simulink model "simF16_nlinplant_unmatched"  (R2020a)
settings: Solver=ode14x  StartTime=0  StopTime=sim_t  FixedStep=Ts  RelTol=1e-3  EnableMultiTasking=on
values from neighbouring files (symbols this model uses):
  adapt_gain_no_Bm = -inv(Phi)*Mat_expm    [main_f16.m]
  Alti = A([3,5],[3,5])    [main_f16.m]
  alti_0 = sim_scenarios{i}(1)    [main_f16.m]
  altitudes = [5000 5000 5000 5000 5000 5000 5000 5000 5000 5000 5000 5000 ... (96 elements, 12x8)]    [lpv_model.mat]    (also in parameters_twoparas_ss_large_omega_range.mat)
  Ap0 = [-0.965786131048  0.940676857343; -3.44113853073  -1.30180201506]    [lpv_model.mat]    (also in parameters_twoparas_ss_large_omega_range.mat)
  Ap1 = [-0.695446741137  -0.0219021350224; -2.98749239517  -0.883673052084]    [lpv_model.mat]    (also in parameters_twoparas_ss_large_omega_range.mat)
  Ap2 = [-0.00376589285085  -0.000767161245953; 0.0864223450734  -0.00373090940113]    [lpv_model.mat]    (also in parameters_twoparas_ss_large_omega_range.mat)
  Blti = B([3,5],2)    [main_f16.m]
  Bp0 = [-0.00202220767716 -0.26458627897]    [lpv_model.mat]    (also in parameters_twoparas_ss_large_omega_range.mat)
  Bp1 = [-0.00144075289053 -0.241352628281]    [lpv_model.mat]    (also in parameters_twoparas_ss_large_omega_range.mat)
  Bp2 = [-6.1325666296e-07 -0.000135209280723]    [lpv_model.mat]    (also in parameters_twoparas_ss_large_omega_range.mat)
  control_trims = [0.149023636522 -3.3718875614 -3.81812148762e-13 -1.65140410369e-12 0.145229850722 -2.69024444853 -5.03470498061e-14 -2.84198247296e-13 0.146487538342 -2.32267253452 7.51716315972e-14 5.14334939656e-13 ... (384 elements, 4x12x8)]    [lpv_model.mat]    (also in parameters_twoparas_ss_large_omega_range.mat)
  Cp = [1 0]    [lpv_model.mat]    (also in parameters_twoparas_ss_large_omega_range.mat)
  duration = 3.01    [main_f16.m]
  enable_L1 = 1    [main_f16.m]
  enable_um_dist_comp = 1    [main_f16.m]
  L = [-1.0529546208e-07 9.01402394984e-07 -6.3448246624e-08 3.15977865752e-07 2.28928663113e-09 -4.32057794956e-09]    [parameters_twoparas_ss_large_omega_range.mat]
  opt =     [unmatched_comp_filter.mat]
  pbar_lower_bnd = 37.1201390864    [lpv_model.mat]    (also in parameters_twoparas_ss_large_omega_range.mat)
  pbar_upper_bnd = 830.356708228    [lpv_model.mat]    (also in parameters_twoparas_ss_large_omega_range.mat)
  r2d = 180/pi    (= 57.2957795131)    [main_f16.m]
  ref_step = 2    [main_f16.m]
  sample_time = Ts    (= 0.001)    [main_f16.m]
  simu_index = simu_index+1    (= 2)    [main_f16.m]
  state_trims = [350 0.128572104103 1.56844869675e-16 0 0.128572104103 0 0 0 0 0 0 5000 ... (1248 elements, 13x12x8)]    [lpv_model.mat]    (also in parameters_twoparas_ss_large_omega_range.mat)
  Ts = 1e-3    (= 0.001)    [main_f16.m]
  unknown_input_gain = .7    (= 0.7)    [main_f16.m]
  veloc_0 = sim_scenarios{i}(2)    [main_f16.m]
  veloc_max = 900    [lpv_model.mat]    (also in parameters_twoparas_ss_large_omega_range.mat)
  veloc_min = 350    [lpv_model.mat]    (also in parameters_twoparas_ss_large_omega_range.mat)
  velocities = [350 400 450 500 550 600 650 700 750 800 850 900 ... (96 elements, 12x8)]    [lpv_model.mat]    (also in parameters_twoparas_ss_large_omega_range.mat)
  X = [4.80336810738e-09 -1.50779531784e-08 -1.50779531784e-08 7.69063603425e-08 2.19210658353e-09 -1.15520629836e-08 -1.15520629836e-08 6.7948487849e-08 9.47019033424e-11 -1.37129742327e-10 -1.37129742327e-10 2.78905243689e-10]    [parameters_twoparas_ss_large_omega_range.mat]
undefined symbols (not defined in the file or in its folder): C_den, C_num, control_trim, state_trim
settings Model: ExtModeAutoUpdateStatusClock=off  Creator=keviczky  LastModifiedBy=Boran
settings DataIOCC: Decimation=50  SaveFormat=Array  SignalLoggingSaveFormat=ModelDataLogs  ReturnWorkspaceOutputs=off  SignalLoggingName=sigsOut
settings OptimizationCC: BooleanDataType=off
settings DebuggingCC: AlgebraicLoopMsg=error  SaveWithParameterizedLinksMsg=none  UnderspecifiedInitializationDetection=Classic  MergeDetectMultiDrivingBlocksExec=none  SignalResolutionControl=TryResolveAllWithWarning  MultiTaskDSMMsg=warning  MultiTaskCondExecSysMsg=none  ArithmeticOperatorsInVariantConditions=warning
settings HardwareCC: ProdBitPerPointer=32  ProdBitPerSizeT=32  ProdBitPerPtrDiffT=32  ProdLargestAtomicFloat=None  ProdIntDivRoundTo=Undefined  ProdEndianess=Unspecified  ProdWordSize=32  ProdHWDeviceType=32-bit Generic  TargetBitPerPointer=64  TargetBitPerSizeT=64  TargetBitPerPtrDiffT=64  TargetLongLongMode=on  TargetIntDivRoundTo=Zero  TargetEndianess=LittleEndian  TargetWordSize=64  TargetHWDeviceType=MATLAB Host  ProdEqTarget=off
settings ModelReferenceCC: PropagateSignalLabelsOutOfModel=off
settings SFSimCC: CustomCodeUndefinedFunction=UseInterfaceOnly
settings GRTTargetCC: CombineOutputUpdateFcns=off  GRTInterface=on
settings ConfigComp: CovMetricSettings=dw  CovHtmlReporting=on  CovSaveCumulativeToWorkspaceVar=on  CovSaveSingleToWorkspaceVar=on

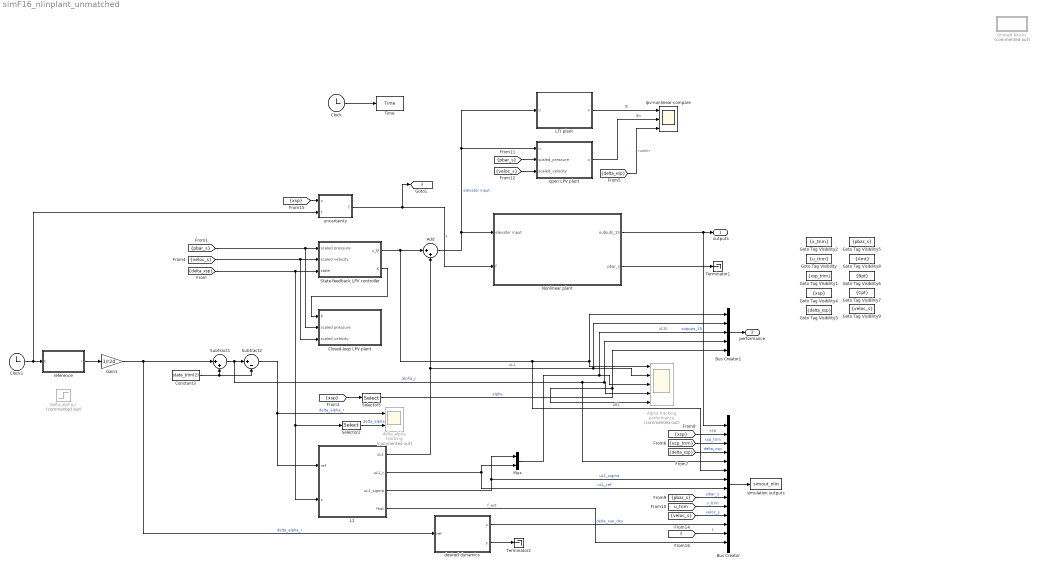
== system simF16_nlinplant_unmatched ==
  Add : Sum  Inputs=|++
  Alpha tracking performance : Scope  Commented=on  NumInputPorts=5
  Bus Creator : BusCreator  Inputs=14
  Bus Creator1 : BusCreator  Inputs=5
  Clock : Clock
      settings: Decimation=50
  Clock1 : Clock
      settings: Decimation=50
  Closed-loop LPV plant : Subsystem
  Constant3 : Constant  Value=state_trim(2)
  Gain1 : Gain  Gain=1/r2d
  Goto Tag Visibility : GotoTagVisibility  GotoTag=u_trim
  Goto Tag Visibility1 : GotoTagVisibility  GotoTag=xsp_trim
  Goto Tag Visibility2 : GotoTagVisibility  GotoTag=x_trim
  Goto Tag Visibility3 : GotoTagVisibility  GotoTag=delta_xsp
  Goto Tag Visibility4 : GotoTagVisibility  GotoTag=xsp
  Goto Tag Visibility5 : GotoTagVisibility  GotoTag=pbar_s
  Goto Tag Visibility6 : GotoTagVisibility  GotoTag=Bpt
  Goto Tag Visibility7 : GotoTagVisibility  GotoTag=Cpt
  Goto Tag Visibility8 : GotoTagVisibility  GotoTag=Amt
  Goto Tag Visibility9 : GotoTagVisibility  GotoTag=veloc_s
  "L1 " : Subsystem
  LTI plant : Subsystem
  Mux : Mux  Inputs=2
  "Nonlinear plant " : Subsystem
  Selector2 : Selector  InputPortWidth=2  IndexOptions=Index vector (dialog)  Indices=1  OutputSizes=1
  Selector5 : Selector  InputPortWidth=2  IndexOptions=Index vector (dialog)  Indices=1  OutputSizes=1
  State-feedback LPV controller : Subsystem
  Subtract1 : Sum  Inputs=|++
  Subtract2 : Sum  Inputs=|+-
  Terminator1 : Terminator
  Terminator2 : Terminator
  Time : ToWorkspace  VariableName=Time  SampleTime=-1
      settings: Decimation=100
  Unused blocks : Subsystem  Commented=on
  delta_alpha tracking : Scope  Commented=on  NumInputPorts=2
  delta_alpha_r : Step  Commented=on  SampleTime=0
  desired dynamics : Subsystem
  lpv-nonlinear-compare : Scope  NumInputPorts=3
  open LPV plant : Subsystem
  reference : MATLAB Function  TreatAsAtomicUnit=on
  simulation outputs : ToWorkspace  VariableName=simout_nlin  SaveFormat=Timeseries  SampleTime=-1
      settings: Decimation=2
  uncertainty : MATLAB Function  TreatAsAtomicUnit=on
  outputs : Outport  VectorParamsAs1DForOutWhenUnconnected=off
  performance : Outport  Port=2  VectorParamsAs1DForOutWhenUnconnected=off
  tag scope: f=global
  wires:
  Clock/1 -> Time/1
  "L1 "/4(fhat) -> Bus Creator/14  "f_est"
  [f] -> Bus Creator/13  "f"
  [delta_xsp] -> lpv-nonlinear-compare/3  "nonlin"
  uncertainty/1(f) -> "Nonlinear plant "/2(f), [f]  "f"
  open LPV plant/1(x) -> lpv-nonlinear-compare/2  "lpv"
  [pbar_s] -> open LPV plant/2(scaled_pressure)
  [delta_xsp] -> Bus Creator/4  "delta_xsp"
  Add/1 -> "Nonlinear plant "/1(elevator input), LTI plant/1(u), open LPV plant/1(u)  "elevator input"
  Clock1/1 -> uncertainty/2(t), reference/1(t)
  Bus Creator1/1 -> performance/1
  [xsp] -> uncertainty/1(x)
  desired dynamics/1(x) -> Bus Creator/12  "delta_xsp_des"
  desired dynamics/2(y) -> Terminator2/1
  [veloc_s] -> Bus Creator/11  "veloc_s"
  [xsp] -> Bus Creator/2  "xsp"
  State-feedback LPV controller/2(K) -> Closed-loop LPV plant/1(K)
  "Nonlinear plant "/1(outputs_15) -> outputs/1, Bus Creator/1  "outputs_15"
  Gain1/1 -> desired dynamics/1(ref), Subtract1/1  "delta_alpha_r"
  [veloc_s] -> open LPV plant/3(scaled_velocity)
  [xsp_trim] -> Bus Creator/3  "xsp_trim"
  LTI plant/1(x) -> lpv-nonlinear-compare/1  "lti"
  reference/1(r) -> Gain1/1
  [delta_xsp] -> State-feedback LPV controller/3(state), "L1 "/2(x), Selector2/1
  "L1 "/2(uL1_r) -> Mux/2, Bus Creator/8  "uL1_ref"
  [veloc_s] -> Closed-loop LPV plant/3(scaled velocity), State-feedback LPV controller/2(scaled velocity)
  [xsp] -> Selector5/1
  Selector2/1 -> delta_alpha tracking/2  "delta_alpha"
  Constant3/1 -> Subtract2/2, Subtract1/2
  "L1 "/1(uL1) -> Add/2, Bus Creator1/2, Alpha tracking performance/2  "uL1"
  [pbar_s] -> Bus Creator/9  "pbar_s"
  Bus Creator/1 -> simulation outputs/1
  State-feedback LPV controller/1(u_bl) -> Add/1, Bus Creator/6, Bus Creator1/1, Alpha tracking performance/1  "uBL"
  "L1 "/3(uL1_sigma) -> Mux/1, Bus Creator/7  "uL1_sigma"
  Subtract2/1 -> "L1 "/1(ref), delta_alpha tracking/1  "delta_alpha_r"
  [pbar_s] -> Closed-loop LPV plant/2(scaled pressure), State-feedback LPV controller/1(scaled pressure)
  Mux/1 -> Bus Creator1/3, Alpha tracking performance/3  "uL1s"
  Selector5/1 -> Alpha tracking performance/5, Bus Creator1/5  "alpha"
  "Nonlinear plant "/2(pbar_s) -> Terminator1/1
  Subtract1/1 -> Alpha tracking performance/4, Bus Creator1/4, Bus Creator/5, Subtract2/1  "alpha_r"
  [u_trim] -> Bus Creator/10  "u_trim"

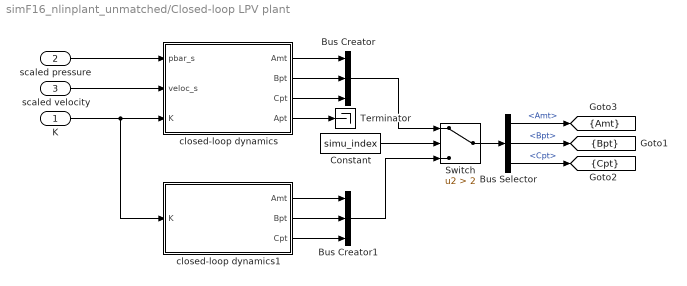
== system simF16_nlinplant_unmatched/Closed-loop LPV plant ==
  K : Inport
  scaled pressure : Inport  Port=2
  scaled velocity : Inport  Port=3
  Bus Creator : BusCreator  Inputs=3
  Bus Creator1 : BusCreator  Inputs=3
  Bus Selector : BusSelector  OutputSignals=Amt,Bpt,Cpt
  Constant : Constant  Value=simu_index
  Switch : Switch  Criteria=u2 > Threshold  Threshold=2
  Terminator : Terminator
  closed-loop dynamics : MATLAB Function  TreatAsAtomicUnit=on
  closed-loop dynamics1 : MATLAB Function  TreatAsAtomicUnit=on
  tag scope: Amt=scoped, Bpt=scoped, Cpt=scoped
  wires:
  scaled pressure/1 -> closed-loop dynamics/1(pbar_s)
  scaled velocity/1 -> closed-loop dynamics/2(veloc_s)
  closed-loop dynamics/2(Bpt) -> Bus Creator/2
  closed-loop dynamics/4(Apt) -> Terminator/1
  closed-loop dynamics/1(Amt) -> Bus Creator/1
  closed-loop dynamics/3(Cpt) -> Bus Creator/3
  closed-loop dynamics1/1(Amt) -> Bus Creator1/1
  closed-loop dynamics1/2(Bpt) -> Bus Creator1/2
  closed-loop dynamics1/3(Cpt) -> Bus Creator1/3
  Bus Creator/1 -> Switch/1
  Bus Creator1/1 -> Switch/3
  Switch/1 -> Bus Selector/1
  Bus Selector/1 -> [Amt]  "<Amt>"
  Bus Selector/2 -> [Bpt]  "<Bpt>"
  Bus Selector/3 -> [Cpt]  "<Cpt>"
  K/1 -> closed-loop dynamics1/1(K), closed-loop dynamics/3(K)
  Constant/1 -> Switch/2

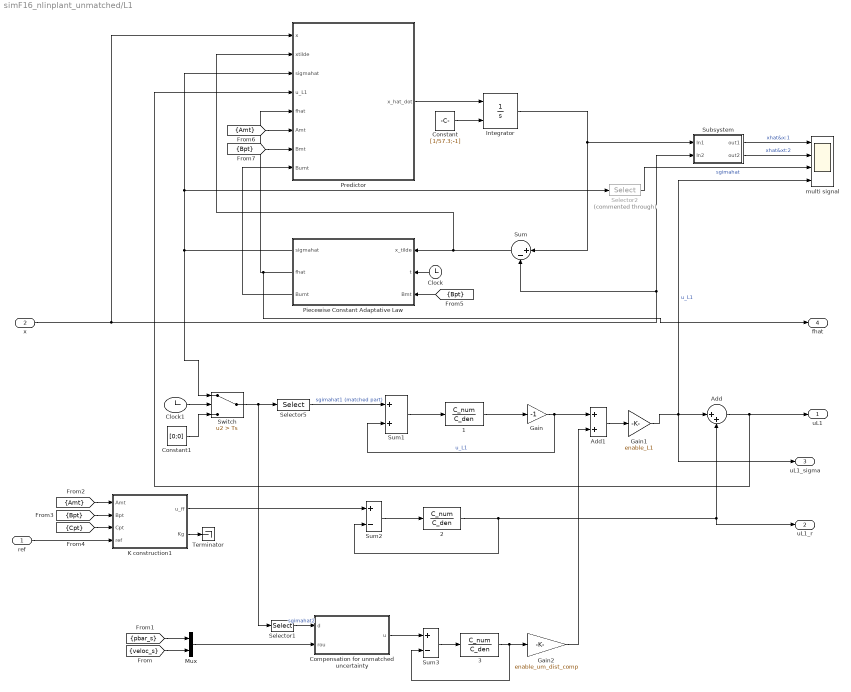
== system simF16_nlinplant_unmatched/L1  ==
  ref : Inport
  x : Inport  Port=2
  " 1" : TransferFcn  Numerator=C_num  Denominator=C_den
  " 2" : TransferFcn  Numerator=C_num  Denominator=C_den
  " 3" : TransferFcn  Numerator=C_num  Denominator=C_den
  Add : Sum  Inputs=|++
  Add1 : Sum
  Clock : Clock
  Clock1 : Clock
      settings: Decimation=50
  Compensation for unmatched uncertainty : Subsystem
  Constant : Constant  Value=[1/57.3;-1]
  Constant1 : Constant  Value=[0;0]
  Gain : Gain  Gain=-1
  Gain1 : Gain  Gain=enable_L1
  Gain2 : Gain  Gain=enable_um_dist_comp
  Integrator : Integrator  InitialConditionSource=external
  K construction1 : MATLAB Function  TreatAsAtomicUnit=on
  Mux : Mux  Inputs=2
  Piecewise Constant Adaptative Law : MATLAB Function  TreatAsAtomicUnit=on
  Predictor : MATLAB Function  TreatAsAtomicUnit=on
  Selector1 : Selector  InputPortWidth=2  IndexOptions=Index vector (dialog)  Indices=2  OutputSizes=1
  Selector2 : Selector  Commented=through  InputPortWidth=2  IndexOptions=Index vector (dialog)  Indices=[1]  OutputSizes=1
  Selector5 : Selector  InputPortWidth=2  IndexOptions=Index vector (dialog)  Indices=[1]  OutputSizes=1
  Subsystem : Subsystem
  Sum : Sum  Inputs=|+-
  Sum1 : Sum
  Sum2 : Sum  Inputs=+-
  Sum3 : Sum  Inputs=+-
  Switch : Switch  Criteria=u2 > Threshold  Threshold=Ts
  Terminator : Terminator
  "multi signal " : Scope  NumInputPorts=4
  uL1 : Outport  VectorParamsAs1DForOutWhenUnconnected=off
  uL1_r : Outport  Port=2  VectorParamsAs1DForOutWhenUnconnected=off
  uL1_sigma : Outport  Port=3  VectorParamsAs1DForOutWhenUnconnected=off
  fhat : Outport  Port=4  VectorParamsAs1DForOutWhenUnconnected=off
  wires:
  Constant/1 -> Integrator/2
  Predictor/1(x_hat_dot) -> Integrator/1
  Integrator/1 -> Sum/1, Subsystem/1(In1)
  Clock/1 -> Piecewise Constant Adaptative Law/2(t)
  x/1 -> Subsystem/2(In2), Sum/2, Predictor/1(x)
  Selector2/1 -> "multi signal "/3  "sgimahat"
  Gain1/1 -> Add/1, uL1_sigma/1, "multi signal "/4  "u_L1"
  " 1"/1 -> Gain/1
  [Cpt] -> K construction1/3(Cpt)
  [Bpt] -> K construction1/2(Bpt)
  " 2"/1 -> Add/2, uL1_r/1, Sum2/2
  ref/1 -> K construction1/4(ref)
  [Amt] -> K construction1/1(Amt)
  [Bpt] -> Piecewise Constant Adaptative Law/3(Bmt)
  [Amt] -> Predictor/6(Amt)
  [Bpt] -> Predictor/7(Bmt)
  Sum/1 -> Piecewise Constant Adaptative Law/1(x_tilde), Predictor/2(xtilde)
  Selector5/1 -> Sum1/1  "sgimahat1 (matched part)"
  Sum1/1 -> " 1"/1
  Piecewise Constant Adaptative Law/3(Bumt) -> Predictor/8(Bumt)
  Sum2/1 -> " 2"/1
  Subsystem/1(out1) -> "multi signal "/1  "xhat&x:1"
  Subsystem/2(out2) -> "multi signal "/2  "xhat&xt:2"
  Add/1 -> Predictor/4(u_L1), uL1/1
  K construction1/2(Kg) -> Terminator/1
  Gain2/1 -> Add1/2
  Mux/1 -> Compensation for unmatched uncertainty/2(rou)
  Selector1/1 -> Compensation for unmatched uncertainty/1(d)  "sgimahat2"
  [veloc_s] -> Mux/2
  Compensation for unmatched uncertainty/1(u) -> Sum3/1
  Sum3/1 -> " 3"/1
  [pbar_s] -> Mux/1
  " 3"/1 -> Gain2/1, Sum3/2
  Piecewise Constant Adaptative Law/1(sigmahat) -> Switch/1, Predictor/3(sigmahat), Selector2/1
  Add1/1 -> Gain1/1
  Gain/1 -> Sum1/2, Add1/1  "u_L1"
  Piecewise Constant Adaptative Law/2(fhat) -> fhat/1, Predictor/5(fhat)
  Constant1/1 -> Switch/3
  Switch/1 -> Selector1/1, Selector5/1
  Clock1/1 -> Switch/2
  K construction1/1(u_ff) -> Sum2/1

== system simF16_nlinplant_unmatched/LTI plant ==
  u : Inport
  Integrator : Integrator
  K construction : MATLAB Function  TreatAsAtomicUnit=on
  x : Outport  VectorParamsAs1DForOutWhenUnconnected=off
  wires:
  u/1 -> K construction/2(u)
  K construction/1(xdot) -> Integrator/1
  Integrator/1 -> x/1, K construction/1(x)

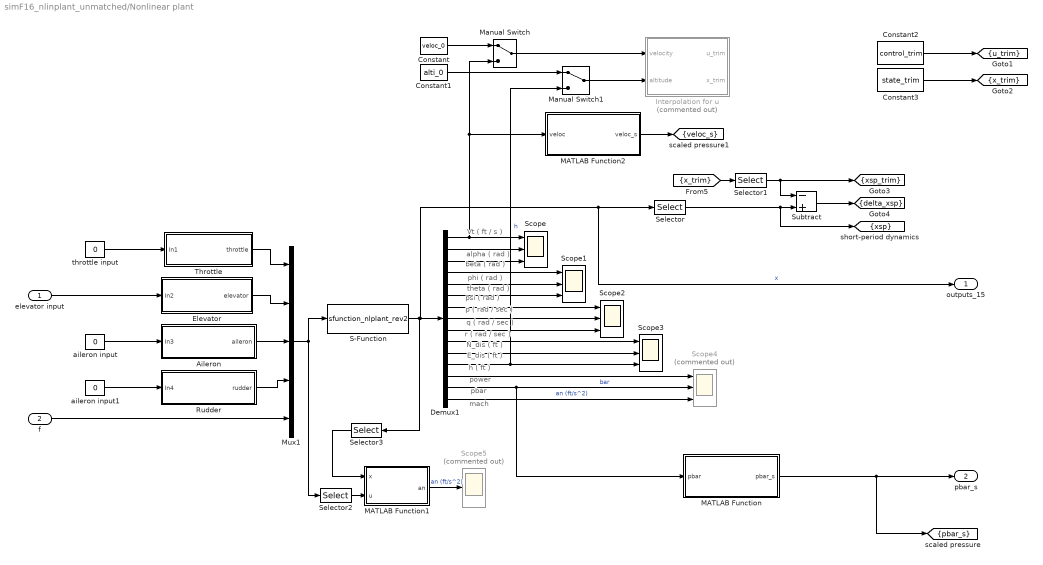
== system simF16_nlinplant_unmatched/Nonlinear plant  ==
  note: Vt ( ft / s )
  note: alpha ( rad )
  note: beta ( rad )
  note: phi ( rad )
  note: theta ( rad )
  note: psi ( rad )
  note: p ( rad / sec )
  note: q ( rad / sec )
  note: r ( rad / sec )
  note: N_dis ( ft )
  note: E_dis ( ft )
  note: h ( ft )
  note: power
  note: pbar
  note: mach
  elevator input : Inport
  f : Inport  Port=2
  Aileron : Subsystem
  Constant : Constant  Value=veloc_0
  Constant1 : Constant  Value=alti_0
  Constant2 : Constant  Value=control_trim
  Constant3 : Constant  Value=state_trim
  Demux1 : Demux  Outputs=15
  Elevator : Subsystem
  Interpolation for u : Subsystem  Commented=on
  MATLAB Function : MATLAB Function  TreatAsAtomicUnit=on
  MATLAB Function1 : MATLAB Function  TreatAsAtomicUnit=on
  MATLAB Function2 : MATLAB Function  TreatAsAtomicUnit=on
  Manual Switch : ManualSwitch
  Manual Switch1 : ManualSwitch
  Mux1 : Mux  Inputs=5
  Rudder : Subsystem
  S-Function : S-Function  FunctionName=sfunction_nlplant_rev2  Parameters="state_trim,  xcg"  SFunctionDeploymentMode=off  EnableBusSupport=off
  Scope{,1..3} (4 alike) : Scope  NumInputPorts=3
  Scope4 : Scope  Commented=on  NumInputPorts=3
  Scope5 : Scope  Commented=on
  Selector : Selector  InputPortWidth=15  IndexOptions=Index vector (dialog)  Indices=[2 8]  OutputSizes=1
  Selector1 : Selector  InputPortWidth=13  IndexOptions=Index vector (dialog)  Indices=[2 8]  OutputSizes=1
  Selector2 : Selector  InputPortWidth=6  IndexOptions=Index vector (dialog)  Indices=1:4  OutputSizes=1
  Selector3 : Selector  InputPortWidth=15  IndexOptions=Index vector (dialog)  Indices=[1:13]  OutputSizes=1
  Subtract : Sum  Inputs=-+
  Throttle : Subsystem
  aileron input : Constant  Value=0
  aileron input1 : Constant  Value=0
  throttle input : Constant  Value=0
  outputs_15 : Outport  VectorParamsAs1DForOutWhenUnconnected=off
  pbar_s : Outport  Port=2  VectorParamsAs1DForOutWhenUnconnected=off
  tag scope: delta_xsp=scoped, pbar_s=scoped, u_trim=scoped, veloc_s=scoped, x_trim=scoped, xsp=scoped, xsp_trim=scoped
  wires:
  Demux1/6 -> Scope1/3
  Demux1/7 -> Scope2/1
  Demux1/2 -> Scope/2
  Constant1/1 -> Manual Switch1/1
  Demux1/3 -> Scope/3
  aileron input1/1 -> Rudder/1(In4)
  S-Function/1 -> Selector3/1, Demux1/1, outputs_15/1, Selector/1  "x"
  Demux1/4 -> Scope1/1
  Demux1/11 -> Scope3/2
  Demux1/8 -> Scope2/2
  Demux1/5 -> Scope1/2
  Selector3/1 -> MATLAB Function1/1(x)
  Elevator/1(elevator) -> Mux1/2
  Demux1/12 -> Scope3/3, Manual Switch1/2  "h"
  aileron input/1 -> Aileron/1(In3)
  Throttle/1(throttle) -> Mux1/1
  Selector1/1 -> [xsp_trim], Subtract/1
  throttle input/1 -> Throttle/1(In1)
  Manual Switch1/1 -> Interpolation for u/2(altitude)
  Selector/1 -> [xsp], Subtract/2
  Mux1/1 -> S-Function/1, Selector2/1
  Demux1/10 -> Scope3/1
  Subtract/1 -> [delta_xsp]
  Demux1/9 -> Scope2/3
  elevator input/1 -> Elevator/1(In2)
  Manual Switch/1 -> Interpolation for u/1(velocity)
  Demux1/13 -> Scope4/1
  Aileron/1(aileron) -> Mux1/3
  MATLAB Function1/1(an) -> Scope5/1  "an (ft/s^2)"
  Rudder/1(rudder) -> Mux1/4
  Demux1/1 -> MATLAB Function2/1(veloc), Manual Switch/2, Scope/1
  Demux1/15 -> Scope4/3  "an (ft/s^2)"
  Demux1/14 -> MATLAB Function/1(pbar), Scope4/2  "bar"
  [x_trim] -> Selector1/1
  Constant/1 -> Manual Switch/1
  MATLAB Function/1(pbar_s) -> pbar_s/1, [pbar_s]
  MATLAB Function2/1(veloc_s) -> [veloc_s]
  Constant2/1 -> [u_trim]
  Constant3/1 -> [x_trim]
  f/1 -> Mux1/5
  Selector2/1 -> MATLAB Function1/2(u)

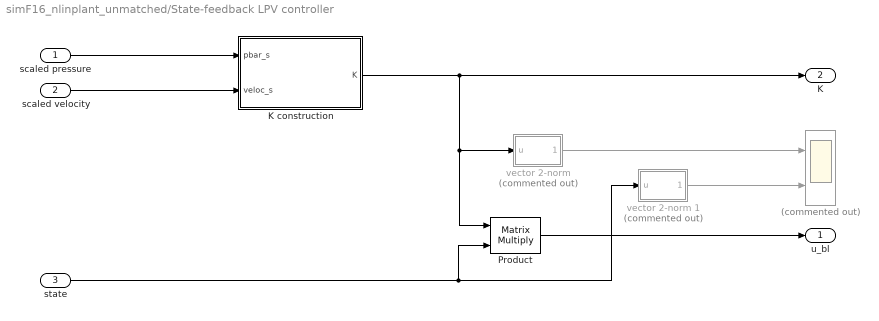
== system simF16_nlinplant_unmatched/State-feedback LPV controller ==
  scaled pressure : Inport
  scaled velocity : Inport  Port=2
  state : Inport  Port=3
  " " : Scope  Commented=on  NumInputPorts=2
  K construction : MATLAB Function  TreatAsAtomicUnit=on
  Product : Product  Multiplication=Matrix(*)
  "vector 2-norm " : Subsystem  Commented=on
  vector 2-norm 1 : Subsystem  Commented=on
  u_bl : Outport  VectorParamsAs1DForOutWhenUnconnected=off
  K : Outport  Port=2  VectorParamsAs1DForOutWhenUnconnected=off
  wires:
  scaled pressure/1 -> K construction/1(pbar_s)
  K construction/1(K) -> "vector 2-norm "/1(u), Product/1, K/1
  "vector 2-norm "/1(||u||_2) -> " "/1
  vector 2-norm 1/1(||u||_2) -> " "/2
  state/1 -> Product/2, vector 2-norm 1/1(u)
  Product/1 -> u_bl/1
  scaled velocity/1 -> K construction/2(veloc_s)

== system simF16_nlinplant_unmatched/Unused blocks ==
  From4 : From  Commented=on  GotoTag=pbar_s  TagVisibility=global
  Goto7 : Goto  Commented=on  GotoTag=u_trim  TagVisibility=global
  Goto8 : Goto  Commented=on  GotoTag=x_trim  TagVisibility=global
  Interpolation for u0 : Subsystem  Commented=on
  Interpolation for u5 : Subsystem  Commented=on
  Interpolation for x0 : Subsystem  Commented=on
  MATLAB Function : MATLAB Function  TreatAsAtomicUnit=on
  wires:
  ? -> Interpolation for u0/1(pbar)
  Interpolation for u0/1(u0) -> ?  "u0"
  Interpolation for x0/1(x0) -> ?
  Interpolation for u5/1(u_trim) -> Goto7/1
  Interpolation for u5/2(x_trim) -> Goto8/1
  From4/1 -> Interpolation for u5/1(pbar_s)

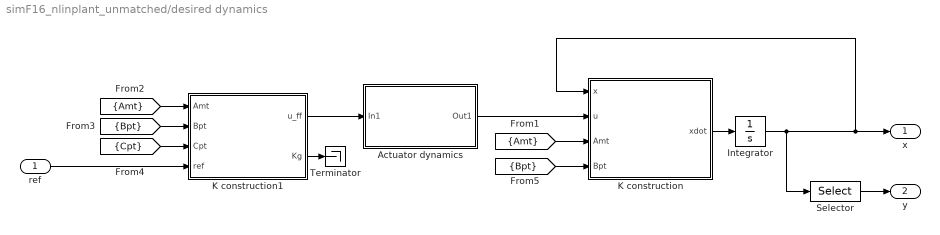
== system simF16_nlinplant_unmatched/desired dynamics ==
  ref : Inport
  Actuator dynamics : Subsystem
  Integrator : Integrator
  K construction : MATLAB Function  TreatAsAtomicUnit=on
  K construction1 : MATLAB Function  TreatAsAtomicUnit=on
  Selector : Selector  InputPortWidth=2  IndexOptions=Index vector (dialog)  Indices=1  OutputSizes=1
  Terminator : Terminator
  x : Outport  VectorParamsAs1DForOutWhenUnconnected=off
  y : Outport  Port=2  VectorParamsAs1DForOutWhenUnconnected=off
  wires:
  K construction1/2(Kg) -> Terminator/1
  [Bpt] -> K construction1/2(Bpt)
  [Amt] -> K construction1/1(Amt)
  K construction1/1(u_ff) -> Actuator dynamics/1(In1)
  ref/1 -> K construction1/4(ref)
  [Cpt] -> K construction1/3(Cpt)
  Integrator/1 -> Selector/1, x/1, K construction/1(x)
  K construction/1(xdot) -> Integrator/1
  [Amt] -> K construction/3(Amt)
  [Bpt] -> K construction/4(Bpt)
  Selector/1 -> y/1
  Actuator dynamics/1(Out1) -> K construction/2(u)

== system simF16_nlinplant_unmatched/open LPV plant ==
  u : Inport
  scaled_pressure : Inport  Port=2
  scaled_velocity : Inport  Port=3
  Integrator : Integrator
  K construction : MATLAB Function  TreatAsAtomicUnit=on
  x : Outport  VectorParamsAs1DForOutWhenUnconnected=off
  wires:
  scaled_pressure/1 -> K construction/3(pbar_s)
  u/1 -> K construction/2(u)
  K construction/1(xdot) -> Integrator/1
  Integrator/1 -> x/1, K construction/1(x)
  scaled_velocity/1 -> K construction/4(veloc_s)

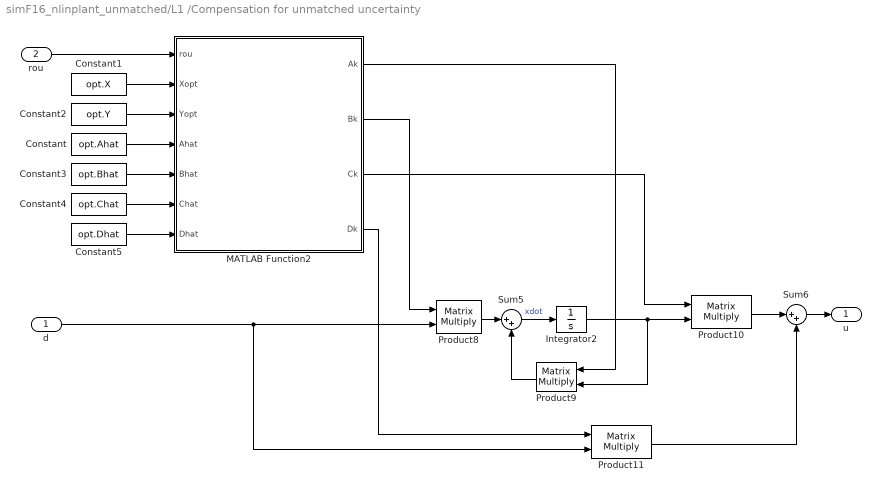
== system simF16_nlinplant_unmatched/L1 /Compensation for unmatched uncertainty ==
  d : Inport
  rou : Inport  Port=2
  Constant : Constant  Value=opt.Ahat  VectorParams1D=off
  Constant1 : Constant  Value=opt.X  VectorParams1D=off
  Constant2 : Constant  Value=opt.Y  VectorParams1D=off
  Constant3 : Constant  Value=opt.Bhat  VectorParams1D=off
  Constant4 : Constant  Value=opt.Chat  VectorParams1D=off
  Constant5 : Constant  Value=opt.Dhat  VectorParams1D=off
  Integrator2 : Integrator
  MATLAB Function2 : MATLAB Function  TreatAsAtomicUnit=on
  Product{8..11} (4 alike) : Product  Multiplication=Matrix(*)
  Sum5 : Sum  Inputs=|++
  Sum6 : Sum  Inputs=|++
  u : Outport  VectorParamsAs1DForOutWhenUnconnected=off
  wires:
  d/1 -> Product8/2, Product11/2
  Sum5/1 -> Integrator2/1  "xdot"
  Product8/1 -> Sum5/1
  Product11/1 -> Sum6/2
  Product10/1 -> Sum6/1
  Integrator2/1 -> Product10/2, Product9/2
  Product9/1 -> Sum5/2
  rou/1 -> MATLAB Function2/1(rou)
  Constant/1 -> MATLAB Function2/4(Ahat)
  Sum6/1 -> u/1
  MATLAB Function2/4(Dk) -> Product11/1
  MATLAB Function2/3(Ck) -> Product10/1
  Constant4/1 -> MATLAB Function2/6(Chat)
  Constant3/1 -> MATLAB Function2/5(Bhat)
  Constant1/1 -> MATLAB Function2/2(Xopt)
  Constant2/1 -> MATLAB Function2/3(Yopt)
  MATLAB Function2/2(Bk) -> Product8/1
  Constant5/1 -> MATLAB Function2/7(Dhat)
  MATLAB Function2/1(Ak) -> Product9/1

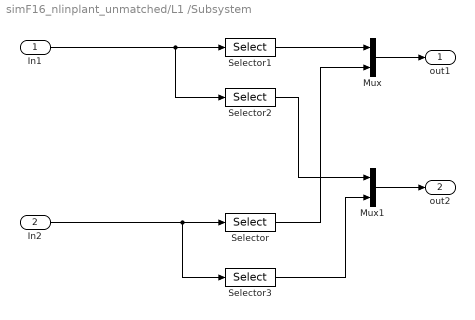
== system simF16_nlinplant_unmatched/L1 /Subsystem ==
  In1 : Inport
  In2 : Inport  Port=2
  Mux : Mux  Inputs=2
  Mux1 : Mux  Inputs=2
  Selector : Selector  InputPortWidth=2  IndexOptions=Index vector (dialog)  Indices=[1]  OutputSizes=1
  Selector1 : Selector  InputPortWidth=2  IndexOptions=Index vector (dialog)  Indices=[1]  OutputSizes=1
  Selector2 : Selector  InputPortWidth=2  IndexOptions=Index vector (dialog)  Indices=2  OutputSizes=1
  Selector3 : Selector  InputPortWidth=2  IndexOptions=Index vector (dialog)  Indices=2  OutputSizes=1
  out1 : Outport  VectorParamsAs1DForOutWhenUnconnected=off
  out2 : Outport  Port=2  VectorParamsAs1DForOutWhenUnconnected=off
  wires:
  In1/1 -> Selector2/1, Selector1/1
  In2/1 -> Selector3/1, Selector/1
  Selector/1 -> Mux/2
  Selector1/1 -> Mux/1
  Mux/1 -> out1/1
  Selector2/1 -> Mux1/1
  Selector3/1 -> Mux1/2
  Mux1/1 -> out2/1

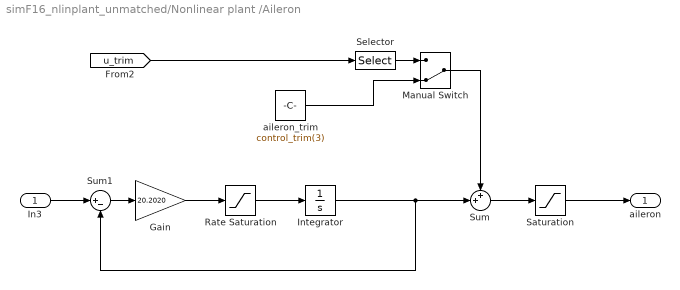
== system simF16_nlinplant_unmatched/Nonlinear plant /Aileron ==
  In3 : Inport
  Gain : Gain  Gain=20.2020  SaturateOnIntegerOverflow=on  OutDataTypeStr=Inherit: Same as input  ParamDataTypeStr=Inherit: Same as input
  Integrator : Integrator  UpperSaturationLimit=21.5  LowerSaturationLimit=-21.5
  Manual Switch : ManualSwitch  CurrentSetting=0
  Rate Saturation : Saturate  UpperLimit=80  LowerLimit=-80
  Saturation : Saturate  UpperLimit=21.5  LowerLimit=-21.5
  Selector : Selector  InputPortWidth=4  IndexOptions=Index vector (dialog)  Indices=3  OutputSizes=1
  Sum : Sum  Inputs=++|  InputSameDT=on  SaturateOnIntegerOverflow=on  OutDataTypeStr=Inherit: Same as first input
  Sum1 : Sum  Inputs=|+-  InputSameDT=on  SaturateOnIntegerOverflow=on  OutDataTypeStr=Inherit: Same as first input
  aileron_trim : Constant  Value=control_trim(3)
  aileron : Outport  VectorParamsAs1DForOutWhenUnconnected=off
  wires:
  In3/1 -> Sum1/1
  Sum1/1 -> Gain/1
  Gain/1 -> Rate Saturation/1
  Rate Saturation/1 -> Integrator/1
  Integrator/1 -> Sum1/2, Sum/2
  Sum/1 -> Saturation/1
  Saturation/1 -> aileron/1
  Selector/1 -> Manual Switch/1
  aileron_trim/1 -> Manual Switch/2
  [u_trim] -> Selector/1
  Manual Switch/1 -> Sum/1

== system simF16_nlinplant_unmatched/Nonlinear plant /Elevator ==
  In2 : Inport
  Actuator dynamics : Subsystem
  Gain1 : Gain  Gain=unknown_input_gain  SaturateOnIntegerOverflow=on  OutDataTypeStr=Inherit: Same as input  ParamDataTypeStr=Inherit: Same as input
  Manual Switch : ManualSwitch  CurrentSetting=0
  Saturation : Saturate  UpperLimit=25  LowerLimit=-25
  Selector : Selector  InputPortWidth=4  IndexOptions=Index vector (dialog)  Indices=2  OutputSizes=1
  Sum : Sum  Inputs=++|  InputSameDT=on  SaturateOnIntegerOverflow=on  OutDataTypeStr=Inherit: Same as first input
  elevator_trim : Constant  Value=control_trim(2)
  elevator : Outport  VectorParamsAs1DForOutWhenUnconnected=off
  wires:
  Sum/1 -> Gain1/1
  Saturation/1 -> elevator/1
  [u_trim] -> Selector/1
  Selector/1 -> Manual Switch/1
  elevator_trim/1 -> Manual Switch/2
  Manual Switch/1 -> Sum/1
  Gain1/1 -> Saturation/1
  In2/1 -> Actuator dynamics/1(In1)
  Actuator dynamics/1(Out1) -> Sum/2

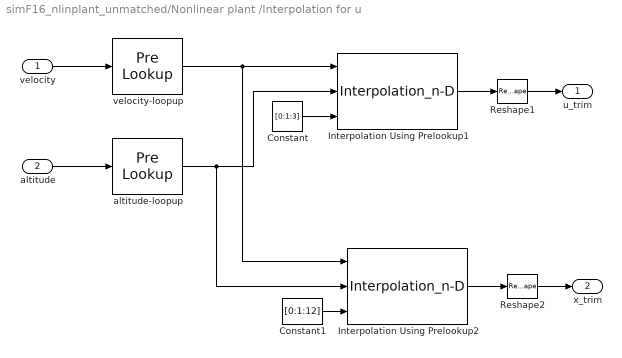
== system simF16_nlinplant_unmatched/Nonlinear plant /Interpolation for u ==
  velocity : Inport
  altitude : Inport  Port=2
  Constant : Constant  Value=[0:1:3]
  Constant1 : Constant  Value=[0:1:12]
  Interpolation Using Prelookup1 : Interpolation_n-D  NumberOfTableDimensions=3  Table=permute( control_trims,[2 3 1])  RequireIndexFractionAsBus=on  NumSelectionDims=1  InternalRulePriority=Speed
      settings: InputPortMap=u0,u1,u2
  Interpolation Using Prelookup2 : Interpolation_n-D  NumberOfTableDimensions=3  Table=permute(state_trims,[2 3 1])  RequireIndexFractionAsBus=on  NumSelectionDims=1  InternalRulePriority=Speed
      settings: InputPortMap=u0,u1,u2
  Reshape1 : Reshape
  Reshape2 : Reshape
  altitude-loopup : PreLookup  BreakpointsData=altitudes(1,:)  OutputSelection=Index and fraction as bus  ExtrapMethod=Linear
  velocity-loopup : PreLookup  BreakpointsData=velocities(:,1)  OutputSelection=Index and fraction as bus  ExtrapMethod=Linear
  u_trim : Outport  VectorParamsAs1DForOutWhenUnconnected=off
  x_trim : Outport  Port=2  VectorParamsAs1DForOutWhenUnconnected=off
  wires:
  Interpolation Using Prelookup1/1 -> Reshape1/1
  Constant/1 -> Interpolation Using Prelookup1/3
  Reshape1/1 -> u_trim/1
  velocity/1 -> velocity-loopup/1
  altitude/1 -> altitude-loopup/1
  altitude-loopup/1 -> Interpolation Using Prelookup2/2, Interpolation Using Prelookup1/2
  Interpolation Using Prelookup2/1 -> Reshape2/1
  Reshape2/1 -> x_trim/1
  velocity-loopup/1 -> Interpolation Using Prelookup2/1, Interpolation Using Prelookup1/1
  Constant1/1 -> Interpolation Using Prelookup2/3

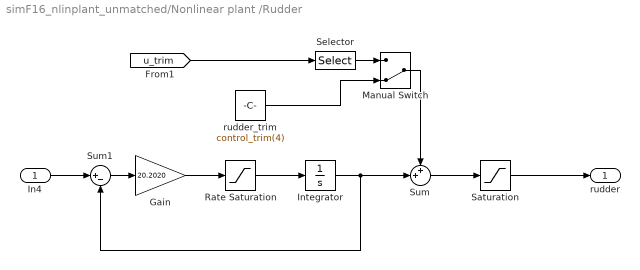
== system simF16_nlinplant_unmatched/Nonlinear plant /Rudder ==
  In4 : Inport
  Gain : Gain  Gain=20.2020  SaturateOnIntegerOverflow=on  OutDataTypeStr=Inherit: Same as input  ParamDataTypeStr=Inherit: Same as input
  Integrator : Integrator  UpperSaturationLimit=30  LowerSaturationLimit=-30
  Manual Switch : ManualSwitch  CurrentSetting=0
  Rate Saturation : Saturate  UpperLimit=120  LowerLimit=-120
  Saturation : Saturate  UpperLimit=30  LowerLimit=-30
  Selector : Selector  InputPortWidth=4  IndexOptions=Index vector (dialog)  Indices=4  OutputSizes=1
  Sum : Sum  Inputs=++|  InputSameDT=on  SaturateOnIntegerOverflow=on  OutDataTypeStr=Inherit: Same as first input
  Sum1 : Sum  Inputs=|+-  InputSameDT=on  SaturateOnIntegerOverflow=on  OutDataTypeStr=Inherit: Same as first input
  rudder_trim : Constant  Value=control_trim(4)
  rudder : Outport  VectorParamsAs1DForOutWhenUnconnected=off
  wires:
  In4/1 -> Sum1/1
  Sum1/1 -> Gain/1
  Gain/1 -> Rate Saturation/1
  Rate Saturation/1 -> Integrator/1
  Integrator/1 -> Sum1/2, Sum/2
  Saturation/1 -> rudder/1
  Sum/1 -> Saturation/1
  Selector/1 -> Manual Switch/1
  rudder_trim/1 -> Manual Switch/2
  [u_trim] -> Selector/1
  Manual Switch/1 -> Sum/1

== system simF16_nlinplant_unmatched/Nonlinear plant /Throttle ==
  In1 : Inport
  Manual Switch : ManualSwitch  CurrentSetting=0
  Saturation : Saturate  UpperLimit=1  LowerLimit=0
  Selector : Selector  InputPortWidth=4  IndexOptions=Index vector (dialog)  Indices=1  OutputSizes=1
  Sum : Sum  InputSameDT=on  SaturateOnIntegerOverflow=on  OutDataTypeStr=Inherit: Same as first input
  throttle_trim : Constant  Value=control_trim(1)
  throttle : Outport  VectorParamsAs1DForOutWhenUnconnected=off
  wires:
  Manual Switch/1 -> Sum/1
  In1/1 -> Sum/2
  Sum/1 -> Saturation/1
  Saturation/1 -> throttle/1
  throttle_trim/1 -> Manual Switch/2
  Selector/1 -> Manual Switch/1
  [u_trim] -> Selector/1

== system simF16_nlinplant_unmatched/State-feedback LPV controller/vector 2-norm  ==
  u : Inport
  Math Function : Math  Operator=square  SignedPower=on  SaturateOnIntegerOverflow=on
  Sqrt : Sqrt  SaturateOnIntegerOverflow=on
  Sum of Elements : Sum  Inputs=+
  ||u||_2 : Outport  VectorParamsAs1DForOutWhenUnconnected=off
  wires:
  Sqrt/1 -> ||u||_2/1
  Math Function/1 -> Sum of Elements/1
  Sum of Elements/1 -> Sqrt/1
  u/1 -> Math Function/1

== system simF16_nlinplant_unmatched/State-feedback LPV controller/vector 2-norm 1 ==
  u : Inport
  Math Function : Math  Operator=square  SignedPower=on  SaturateOnIntegerOverflow=on
  Sqrt : Sqrt  SaturateOnIntegerOverflow=on
  Sum of Elements : Sum  Inputs=+
  ||u||_2 : Outport  VectorParamsAs1DForOutWhenUnconnected=off
  wires:
  u/1 -> Math Function/1
  Sum of Elements/1 -> Sqrt/1
  Math Function/1 -> Sum of Elements/1
  Sqrt/1 -> ||u||_2/1

== system simF16_nlinplant_unmatched/Unused blocks/Interpolation for u0 ==
  pbar : Inport
  Constant : Constant  Value=[0:1:3]
  Interpolation Using Prelookup1 : Interpolation_n-D  Table=control_trims'  RequireIndexFractionAsBus=on  NumSelectionDims=1  InternalRulePriority=Speed
      settings: InputPortMap=u0,u1
  Prelookup1 : PreLookup  BreakpointsData=pbar_vec'  OutputSelection=Index and fraction as bus  ExtrapMethod=Linear
  Reshape1 : Reshape
  u0 : Outport  VectorParamsAs1DForOutWhenUnconnected=off
  wires:
  Prelookup1/1 -> Interpolation Using Prelookup1/1
  pbar/1 -> Prelookup1/1
  Interpolation Using Prelookup1/1 -> Reshape1/1
  Constant/1 -> Interpolation Using Prelookup1/2
  Reshape1/1 -> u0/1

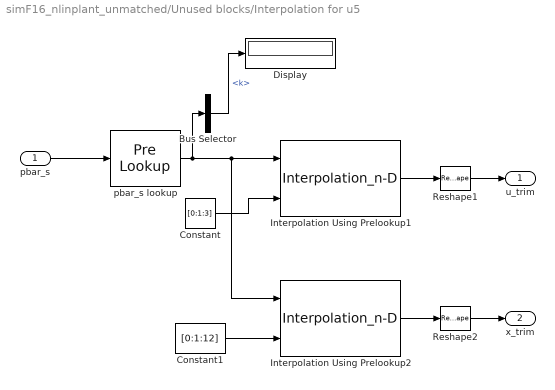
== system simF16_nlinplant_unmatched/Unused blocks/Interpolation for u5 ==
  pbar_s : Inport
  Bus Selector : BusSelector  OutputSignals=k
  Constant : Constant  Value=[0:1:3]
  Constant1 : Constant  Value=[0:1:12]
  Display : Display
  Interpolation Using Prelookup1 : Interpolation_n-D  Table=control_trims_sorted'  RequireIndexFractionAsBus=on  NumSelectionDims=1  InternalRulePriority=Speed
      settings: InputPortMap=u0,u1
  Interpolation Using Prelookup2 : Interpolation_n-D  Table=state_trims_sorted'  RequireIndexFractionAsBus=on  NumSelectionDims=1  InternalRulePriority=Speed
      settings: InputPortMap=u0,u1
  Reshape1 : Reshape
  Reshape2 : Reshape
  pbar_s lookup : PreLookup  BreakpointsData=pbar_svec  OutputSelection=Index and fraction as bus  ExtrapMethod=Linear
  u_trim : Outport  VectorParamsAs1DForOutWhenUnconnected=off
  x_trim : Outport  Port=2  VectorParamsAs1DForOutWhenUnconnected=off
  wires:
  Interpolation Using Prelookup1/1 -> Reshape1/1
  Constant/1 -> Interpolation Using Prelookup1/2
  Reshape1/1 -> u_trim/1
  pbar_s/1 -> pbar_s lookup/1
  Constant1/1 -> Interpolation Using Prelookup2/2
  Reshape2/1 -> x_trim/1
  pbar_s lookup/1 -> Bus Selector/1, Interpolation Using Prelookup2/1, Interpolation Using Prelookup1/1
  Interpolation Using Prelookup2/1 -> Reshape2/1
  Bus Selector/1 -> Display/1  "<k>"

== system simF16_nlinplant_unmatched/Unused blocks/Interpolation for x0 ==
  pbar : Inport
  Constant : Constant  Value=[0:1:12]
  Interpolation Using Prelookup1 : Interpolation_n-D  Table=state_trims'  RequireIndexFractionAsBus=on  NumSelectionDims=1  InternalRulePriority=Speed
      settings: InputPortMap=u0,u1
  Permute Dimensions : PermuteDimensions  Commented=through
  Prelookup1 : PreLookup  BreakpointsData=pbar_vec  OutputSelection=Index and fraction as bus  ExtrapMethod=Linear
  Reshape2 : Reshape
  x0 : Outport  VectorParamsAs1DForOutWhenUnconnected=off
  wires:
  Interpolation Using Prelookup1/1 -> Reshape2/1
  Prelookup1/1 -> Interpolation Using Prelookup1/1
  pbar/1 -> Prelookup1/1
  Permute Dimensions/1 -> x0/1
  Constant/1 -> Interpolation Using Prelookup1/2
  Reshape2/1 -> Permute Dimensions/1

== system simF16_nlinplant_unmatched/desired dynamics/Actuator dynamics ==
  In1 : Inport
  Gain : Gain  Gain=20.2020  SaturateOnIntegerOverflow=on  OutDataTypeStr=Inherit: Same as input  ParamDataTypeStr=Inherit: Same as input
  Integrator : Integrator  UpperSaturationLimit=25  LowerSaturationLimit=-25
  Rate Saturation : Saturate  Commented=through  UpperLimit=60  LowerLimit=-60
  Sum1 : Sum  Inputs=|+-  InputSameDT=on  SaturateOnIntegerOverflow=on  OutDataTypeStr=Inherit: Same as first input
  Out1 : Outport  VectorParamsAs1DForOutWhenUnconnected=off
  wires:
  Sum1/1 -> Gain/1
  Gain/1 -> Rate Saturation/1
  Integrator/1 -> Out1/1, Sum1/2
  Rate Saturation/1 -> Integrator/1
  In1/1 -> Sum1/1

== system simF16_nlinplant_unmatched/Nonlinear plant /Elevator/Actuator dynamics ==
  In1 : Inport
  Gain : Gain  Gain=20.2020  SaturateOnIntegerOverflow=on  OutDataTypeStr=Inherit: Same as input  ParamDataTypeStr=Inherit: Same as input
  Integrator : Integrator  UpperSaturationLimit=25  LowerSaturationLimit=-25
  Rate Saturation : Saturate  Commented=through  UpperLimit=60  LowerLimit=-60
  Sum1 : Sum  Inputs=|+-  InputSameDT=on  SaturateOnIntegerOverflow=on  OutDataTypeStr=Inherit: Same as first input
  Out1 : Outport  VectorParamsAs1DForOutWhenUnconnected=off
  wires:
  Sum1/1 -> Gain/1
  Gain/1 -> Rate Saturation/1
  Integrator/1 -> Out1/1, Sum1/2
  Rate Saturation/1 -> Integrator/1
  In1/1 -> Sum1/1

== matlab function simF16_nlinplant_unmatched/L1 /K construction1 ==
  data: Amt input; u_ff output; Bpt input; Cpt input; ref input; Kg output
function [u_ff,Kg] = feedforward(Amt,Bpt, Cpt,ref)
Kg = -inv(Cpt/Amt*Bpt);
u_ff = Kg*ref;

== matlab function simF16_nlinplant_unmatched/L1 /Piecewise Constant Adaptative Law ==
  settings: updateMethod=DISCRETE
  data: sigmahat output; fhat output; x_tilde input; t input; sample_time parameter; adapt_gain_no_Bm parameter; Bmt input; Bumt output
function [sigmahat, fhat,Bumt]= piecewise_constant(x_tilde,t, sample_time, adapt_gain_no_Bm,Bmt)


% Bumt = null(Bpt); %%%%%%%%%%%%% may need to hard code this to save computational time. 

Bumt = [Bmt(2);-Bmt(1)]; % to satisfy [Bmt Bumt] are full-rank and Bmt'*Bumt = 0


%%%%%%%%%%% up to here
persistent sigmahat_store;
persistent fhat_store;
if isempty(sigmahat_store)
    sigmahat_store = zeros(2,1);
    fhat_store = zeros(2,1);
end

if mod(t,sample_time) == 0   
    
    B = [Bmt Bumt];
%     adapt_gain = B\adapt_gain_no_Bm;
%        
%     sigmahat = adapt_gain*x_tilde;
    fhat = adapt_gain_no_Bm*x_tilde;    
    sigmahat = B\fhat;
    sigmahat_store = sigmahat;
    fhat_store = fhat;
else
    sigmahat = sigmahat_store;
    fhat = fhat_store;
end
% sigmahat = sigmahat(1);  % matched part

== matlab function simF16_nlinplant_unmatched/LTI plant/K construction ==
  data: x input size=2; u input size=1; xdot output size=2; Alti parameter; Blti parameter; unknown_input_gain parameter
function xdot  = LTI_plant(x,u,Alti, Blti,unknown_input_gain)

xdot = Alti*x+Blti*unknown_input_gain*u;

== matlab function simF16_nlinplant_unmatched/open LPV plant/K construction ==
  data: x input size=2; u input size=1; pbar_s input; veloc_s input; xdot output size=2; Ap0 parameter; Bp0 parameter; Ap1 parameter; Bp1 parameter; Ap2 parameter; Bp2 parameter; unknown_input_gain parameter
function xdot  = LPV_plant(x,u,pbar_s,veloc_s,Ap0,Bp0,Ap1,Bp1,Ap2, Bp2,unknown_input_gain)


Bpt = Bp0+pbar_s*Bp1+veloc_s*Bp2;
Apt = Ap0+pbar_s*Ap1+veloc_s*Ap2;
xdot = Apt*x+Bpt*unknown_input_gain*u;

== matlab function simF16_nlinplant_unmatched/reference ==
  data: t input; r output; ref_step parameter; duration parameter
function r = gen_reference(t,ref_step,duration)
%#codegen
if t<=1
    r = 0;
elseif t<= duration+1
    r= ref_step;
else
    r = 0;
end

== matlab function simF16_nlinplant_unmatched/desired dynamics/K construction ==
  data: x input; u input; Amt input; Bpt input; xdot output
function xdot  = LPV_plant(x,u,Amt,Bpt)


xdot = Amt*x+Bpt*u;

== matlab function simF16_nlinplant_unmatched/desired dynamics/K construction1 ==
  data: Amt input; u_ff output; Bpt input; Cpt input; ref input; Kg output
function [u_ff,Kg] = feedforward(Amt,Bpt, Cpt,ref)
Kg = -inv(Cpt/Amt*Bpt);
u_ff = Kg*ref;

== matlab function simF16_nlinplant_unmatched/Nonlinear plant /MATLAB Function2 ==
  data: veloc input; veloc_min parameter; veloc_max parameter; veloc_s output
function veloc_s  = scale_velocity(veloc,veloc_min, veloc_max)
%#codegen

veloc_s = (veloc-veloc_min)/(veloc_max-veloc_min)*2-1;

== matlab function simF16_nlinplant_unmatched/uncertainty ==
  data: x input; t input; f output
function f = fcn(x,t)
%#codegen

% f = sin(2*pi*10*x(1))+cos(2*pi*2*t)+2*sin(2*pi*0.5*t); %10*x(2)^2; 

% f = [0.1*sin(2*pi*10*x(1))+0.1*sin(2*pi*0.5*t); 20*x(2)*x(1)+0.1*cos(2*pi*t)]*0.1; %10*x(2)^2;

f = [0.2*sin(2*pi*10*x(1))+0.1*sin(2*pi*0.5*t); 50*x(2)*x(1)+0.1*cos(2*pi*t)]*.1; %10*x(2)^2;
% f = [0.2*sin(2*pi*10*x(1))+0.2*sin(2*pi*0.5*t); 20*x(2)*x(1)+0.2*cos(2*pi*t)]; %10*x(2)^2; % for 100 rad/s

== matlab function simF16_nlinplant_unmatched/Closed-loop LPV plant/closed-loop dynamics1 ==
  data: Amt output; Bpt output; Cpt output; Alti parameter; Blti parameter; K input
function [Amt,Bpt,Cpt] = get_closed_loop_matrices(Alti, Blti,K)

Bpt = Blti;
Amt = Alti+Bpt*K;
Cpt = [1 0];

== matlab function simF16_nlinplant_unmatched/L1 /Compensation for unmatched uncertainty/MATLAB Function2 ==
  data: rou input; Xopt input; Yopt input; Ak output; Bk output; Ck output; Dk output; Ahat input; Bhat input; Chat input; Dhat input
function [Ak,Bk,Ck,Dk] = Controller(rou,Xopt,Yopt,Ahat,Bhat,Chat,Dhat)
%#codegen
% global Khatopt Xopt Yopt 
Frou = [1 rou(1) rou(2)];
X = Xopt(:,:,1);
Y = Yopt(:,:,1);
Akhat = Ahat(:,:,1);
Bkhat = Bhat(:,:,1);
Ckhat = Chat(:,:,1);
Dkhat = Dhat(:,:,1);

for i=2:length(Frou)
    X = X + Frou(i)*Xopt(:,:,i);
    Y = Y + Frou(i)*Yopt(:,:,i);
    Akhat = Akhat + Frou(i)*Ahat(:,:,i);
    Bkhat = Bkhat + Frou(i)*Bhat(:,:,i);
    Ckhat = Ckhat + Frou(i)*Chat(:,:,i);
    Dkhat = Dkhat + Frou(i)*Dhat(:,:,i);
end

S = X-Y;
Dk = Dkhat;
Bk = Bkhat;
Ck = Ckhat/S;
Ak = Akhat/S;
if max(real(eig(Ak)))>0
   fprintf(1,'controller unstable at theta =[%.3f %.3f]',rou(1),rou(2));
end
end

== matlab function simF16_nlinplant_unmatched/State-feedback LPV controller/K construction ==
  data: pbar_s input; veloc_s input; X parameter; L parameter; K output
function K = CtrlConstr(pbar_s,veloc_s,X,L)
% first order polynomial
Ftheta = [1 pbar_s veloc_s];
Xt = Ftheta(1)*X(:,:,1) + Ftheta(2)*X(:,:,2) + Ftheta(3)*X(:,:,3);
Lt = Ftheta(1)*L(:,:,1) + Ftheta(2)*L(:,:,2) + Ftheta(3)*L(:,:,3);

min_eig = min(real(eig(Xt)));
if min_eig<1e-10
    disp(min_eig);
end
K = Lt/Xt;

== matlab function simF16_nlinplant_unmatched/Nonlinear plant /MATLAB Function ==
  data: pbar input; pbar_lower_bnd parameter; pbar_upper_bnd parameter; pbar_s output
function pbar_s  = scale_pressure(pbar,pbar_lower_bnd, pbar_upper_bnd)
%#codegen

pbar_s = (pbar-pbar_lower_bnd)/(pbar_upper_bnd-pbar_lower_bnd)*2-1;  % scaled dynamic pressure, [-1,1]

== matlab function simF16_nlinplant_unmatched/Closed-loop LPV plant/closed-loop dynamics ==
  data: pbar_s input; veloc_s input; K input; Amt output; Bpt output; Cpt output; Ap0 parameter; Bp0 parameter; Ap1 parameter; Bp1 parameter; Cp parameter; Ap2 parameter; Bp2 parameter; Apt output
function [Amt,Bpt,Cpt,Apt] = LPV_plant(pbar_s,veloc_s,K,Ap0,Bp0,Ap1,Bp1,Cp, Ap2,Bp2)


Bpt = Bp0+pbar_s*Bp1+veloc_s*Bp2;
Apt = Ap0+pbar_s*Ap1+veloc_s*Ap2;
Amt = Apt+Bpt*K;
Cpt = Cp;

== matlab function simF16_nlinplant_unmatched/L1 /Predictor ==
  data: x input; xtilde input; sigmahat input; u_L1 input; fhat input; x_hat_dot output size=2; Atilde parameter; Amt input; Bmt input; Bumt input
function x_hat_dot  = fcn(x, xtilde,sigmahat,u_L1, fhat,Atilde, Amt, Bmt, Bumt)

% x_hat_dot = Amt*x + Bmt*(sigmahat(1)+u_L1)+Bumt*sigmahat(2)+Atilde*xtilde; % note that the nominal input gain is an identity matrix
% x_hat_dot = Amt*x + Bmt*(sigmahat(1)+u_L1)+Atilde*xtilde; % note that the nominal input gain is an identity matrix
x_hat_dot = Amt*x + Bmt*u_L1+Atilde*xtilde+fhat; % note that the nominal input gain is an identity matrix

== matlab function simF16_nlinplant_unmatched/Nonlinear plant /MATLAB Function1 ==
  data: x input double size=13; u input double size=4; an output double size=1
function an = calculate_an(x,u)
s = 300;
cbar = 11.32;
rm = 1.57e-3; % 1 / mass

rtod = 180 / pi; %% radians to degrees
g = 32.174;

%% ---- Assign state variables ---------------
vt = x(1);
alpha = x(2) * rtod; %% x(2) in radians, alpha in degrees.
beta = x(3) * rtod;  %% x(3) in radians, beta in degrees.
q = x(8);
alt = x(12);

%% ---- Look-up tables and component biuldup ------------
el   = u(2);
czt = cz (alpha, beta, el );


[~, ~, ~, ~, qbar, ~] = adc (vt, alt ); 
%% ---- Add damping derivatives ------------
tvt = 0.5 / vt;
cq = cbar * q * tvt;
d = zeros(9,1);
coder.extrinsic('damping')
d = damping( alpha );
czt = czt + cq * d(4);


qs = qbar * s;
rmqs = rm *qs;
az = rmqs * czt;
an = (-1) * az / g;

== matlab function simF16_nlinplant_unmatched/Unused blocks/MATLAB Function ==
  data: alti input; pbar_s output; veloc input; pbar_lower_bnd parameter; pbar_upper_bnd parameter; pbar output
function [pbar_s, pbar] = get_pressure(alti,veloc,pbar_lower_bnd, pbar_upper_bnd)
%#codegen

[pbar_s, pbar] = dynamic_pressue(alti,veloc,pbar_lower_bnd,pbar_upper_bnd);
